simulink model "Spirob_Simulink"  (R2025b)
settings: Solver=VariableStepAuto  StartTime=0.0  StopTime=10  RelTol=1e-3
libraries: mjLib x1
settings Model: Creator=student  LastModifiedBy=student

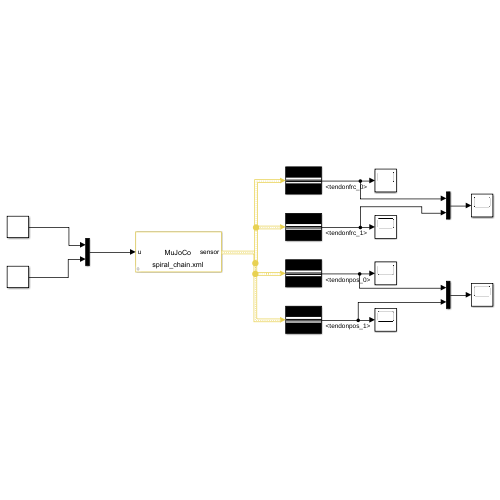
[thumbnail: Simulink's stored preview of the top-level diagram]
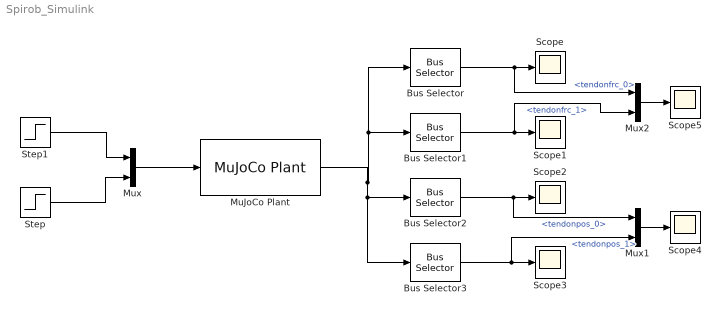
== system Spirob_Simulink ==
  Bus Selector : BusSelector  OutputSignals=tendonfrc_0
  Bus Selector1 : BusSelector  OutputSignals=tendonfrc_1
  Bus Selector2 : BusSelector  OutputSignals=tendonpos_0
  Bus Selector3 : BusSelector  OutputSignals=tendonpos_1
  MuJoCo Plant : mjLib/MuJoCo Plant  controlBus=[]  sensorBus=mj_bus_sensor_7979902499018342666  controlLength=[]  sensorLength=[]  rgbLength=[]  depthLength=[]  sampleTime=0.005  xmlFileRel=/home/student/mujoco_spirob/spiral_chain.xml  xmlFile=/home/student/mujoco_spirob/spiral_chain.xml  renderingType=Global  vsync=off  visualFPS=60  zoomLevel=1  znear=0.0071082  zfar=35.5411  cameraSampleTime=0.020  rgbOutOption=on  depthOutOption=on  controlInterfaceType=Vector
      settings: SourceProductName=MuJoCo Simulator
  Mux : Mux  Inputs=2
  Mux1 : Mux  Inputs=2
  Mux2 : Mux  Inputs=2
  Scope{,1..5} (6 alike) : Scope
      Scope settings: ActiveDisplayYMinimum=-104.38509624641824  ActiveDisplayYMaximum=52.689696943470778
      Scope1 settings: ActiveDisplayYMinimum=-181.25908820458531  ActiveDisplayYMaximum=79.8225820057389
      Scope2 settings: ActiveDisplayYMinimum=-101.16343767438346  ActiveDisplayYMaximum=44.216605499018428  DataLoggingVariableName=ScopeData2
      Scope3 settings: ActiveDisplayYMinimum=-101.16343767438346  ActiveDisplayYMaximum=44.216605499018428  DataLoggingVariableName=ScopeData3
      Scope4 settings: ActiveDisplayYMinimum=0.3724447376139558  ActiveDisplayYMaximum=0.56442459008799239  DataLoggingVariableName=ScopeData4
      Scope5 settings: ActiveDisplayYMinimum=-130.37869889242492  ActiveDisplayYMaximum=81.886012713941255  DataLoggingVariableName=ScopeData5
  Step : Step  After=-20  SampleTime=0
  Step1 : Step  After=0  SampleTime=0
  wires:
  Mux/1 -> MuJoCo Plant/1
  Step/1 -> Mux/2
  Step1/1 -> Mux/1
  MuJoCo Plant/1 -> Bus Selector3/1, Bus Selector2/1, Bus Selector1/1, Bus Selector/1
  Bus Selector/1 -> Mux2/1, Scope/1  "<tendonfrc_0>"
  Bus Selector1/1 -> Mux2/2, Scope1/1  "<tendonfrc_1>"
  Bus Selector2/1 -> Mux1/1, Scope2/1  "<tendonpos_0>"
  Bus Selector3/1 -> Mux1/2, Scope3/1  "<tendonpos_1>"
  Mux1/1 -> Scope4/1
  Mux2/1 -> Scope5/1
